simulink model "sofb_bypass"  (Simulink 7.8)
settings: Solver=VariableStepDiscrete  StartTime=0.0  StopTime=10.0  RelTol=1e-3
values from neighbouring files (symbols this model uses):
  s2ffactor = param.s2ffactor    [simofb.m]
  Ts = param.Ts    [simofb.m]    (also in simofbuvx.m = 0.00032)
settings Model: Creator=danielot  LastModifiedBy=danielot
settings OptimizationCC: InlineParams=on
settings DebuggingCC: AlgebraicLoopMsg=none  ArtificialAlgebraicLoopMsg=none  SolverPrmCheckMsg=none  InheritedTsInSrcMsg=none  DiscreteInheritContinuousMsg=none  TasksWithSamePriorityMsg=none  SigSpecEnsureSampleTimeMsg=none  UnknownTsInhSupMsg=none  ModelReferenceExtraNoncontSigs=none  StateNameClashWarn=none  SimStateInterfaceChecksumMismatchMsg=none

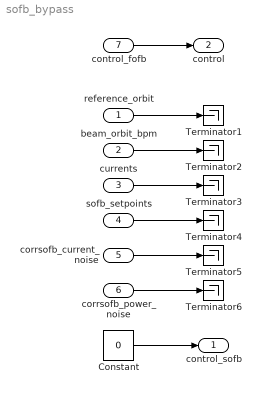
== system sofb_bypass ==
  reference_orbit : Inport  PortDimensions=nbpm  SampleTime=Ts
  beam_orbit_bpm : Inport  Port=2  PortDimensions=nbpm  SampleTime=Ts
  currents : Inport  Port=3  PortDimensions=ncorrmagnet  SampleTime=0
  sofb_setpoints : Inport  Port=4  PortDimensions=ncorrsofb  SampleTime=Ts*s2ffactor
  corrsofb_current_noise : Inport  Port=5  PortDimensions=ncorrsofb  SampleTime=0
  corrsofb_power_noise : Inport  Port=6  PortDimensions=ncorrsofb  SampleTime=0
  control_fofb : Inport  Port=7  PortDimensions=ncorrfofb
  Constant : Constant  Value=0  SampleTime=Ts*s2ffactor
  Terminator{1..6} (6 alike) : Terminator
  control_sofb : Outport
  control : Outport  Port=2
  wires:
  control_fofb/1 -> control/1
  reference_orbit/1 -> Terminator1/1
  corrsofb_power_noise/1 -> Terminator6/1
  corrsofb_current_noise/1 -> Terminator5/1
  sofb_setpoints/1 -> Terminator4/1
  currents/1 -> Terminator3/1
  beam_orbit_bpm/1 -> Terminator2/1
  Constant/1 -> control_sofb/1
